simulink subsystem "bump_mdl"  (R2019b)
settings: Solver=VariableStepAuto  StartTime=0.0  StopTime=10.0  RelTol=1e-3
settings Model: Creator=jingg  LastModifiedBy=jingg

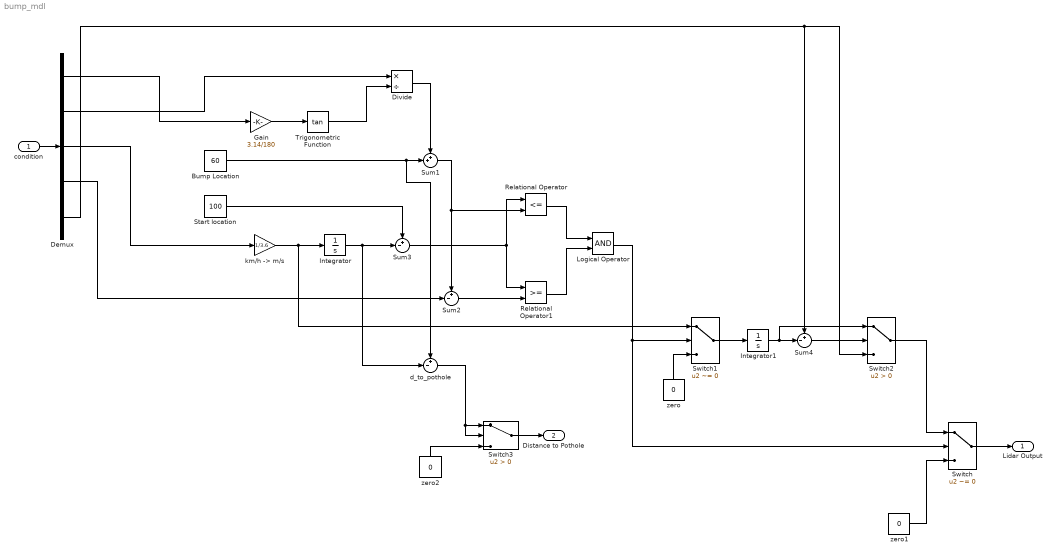
== system bump_mdl ==
  condition : Inport
  Bump Location : Constant  Value=60
  Demux : Demux  Outputs=5
  Divide : Product  Inputs=*/
  Gain : Gain  Gain=3.14/180
  Integrator : Integrator
  Integrator1 : Integrator
  Logical Operator : Logic  AllPortsSameDT=off  OutDataTypeStr=boolean
  Relational Operator : RelationalOperator  Operator=<=  OutDataTypeStr=boolean  RndMeth=Simplest
  Relational Operator1 : RelationalOperator  OutDataTypeStr=boolean  RndMeth=Simplest
  Start location : Constant  Value=100
  Sum1 : Sum  Inputs=++|
  Sum2 : Sum  Inputs=+-|
  Sum3 : Sum  Inputs=+-|
  Sum4 : Sum  Inputs=+-|
  Switch : Switch  Criteria=u2 ~= 0
  Switch1 : Switch  Criteria=u2 ~= 0
  Switch2 : Switch  Criteria=u2 > Threshold
  Switch3 : Switch  Criteria=u2 > Threshold
  Trigonometric Function : Trigonometry  Operator=tan
  d_to_pothole : Sum  Inputs=+-|
  "km/h -> m/s" : Gain  Gain=1/3.6
  zero : Constant  Value=0
  zero1 : Constant  Value=0
  zero2 : Constant  Value=0
  Lidar Output : Outport
  Distance to Pothole : Outport  Port=2
  wires:
  Demux/5 -> Switch2/3, Sum4/1
  Trigonometric Function/1 -> Divide/2
  Sum2/1 -> Relational Operator1/2
  Divide/1 -> Sum1/1
  Demux/4 -> Sum2/2
  Switch/1 -> Lidar Output/1
  Relational Operator1/1 -> Logical Operator/2
  Gain/1 -> Trigonometric Function/1
  zero1/1 -> Switch/3
  Logical Operator/1 -> Switch1/2, Switch/2
  Relational Operator/1 -> Logical Operator/1
  Bump Location/1 -> Sum1/2, d_to_pothole/1
  "km/h -> m/s"/1 -> Integrator/1, Switch1/1
  Sum1/1 -> Relational Operator/2, Sum2/1
  Sum3/1 -> Relational Operator/1, Relational Operator1/1
  Start location/1 -> Sum3/1
  Integrator/1 -> Sum3/2, d_to_pothole/2
  zero/1 -> Switch1/3
  Switch1/1 -> Integrator1/1
  Integrator1/1 -> Sum4/2, Switch2/1
  Sum4/1 -> Switch2/2
  Switch2/1 -> Switch/1
  condition/1 -> Demux/1
  Demux/1 -> Gain/1
  Demux/2 -> Divide/1
  Demux/3 -> "km/h -> m/s"/1
  Switch3/1 -> Distance to Pothole/1
  d_to_pothole/1 -> Switch3/2, Switch3/1
  zero2/1 -> Switch3/3
